simulink library "Chassis_stability_controllers"  (R2024a)
settings: Solver=VariableStepAuto  StartTime=0.0  StopTime=10.0  RelTol=1e-3
undefined symbols (not defined in the file): Ts
settings Model: Creator=Henrique Mesquita  LastModifiedBy=Henrique Mesquita

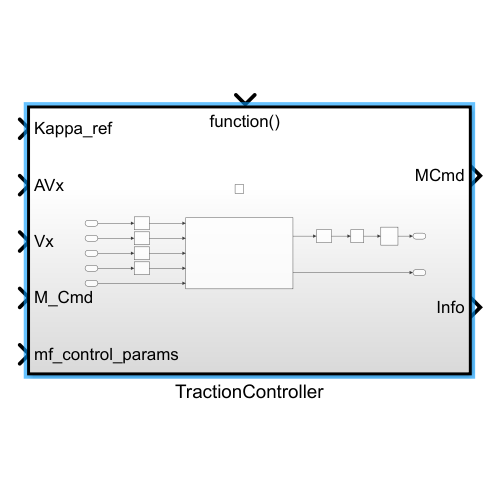
[thumbnail: Simulink's stored preview of the top-level diagram]
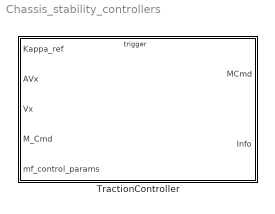
== system Chassis_stability_controllers ==
  TractionController : Subsystem

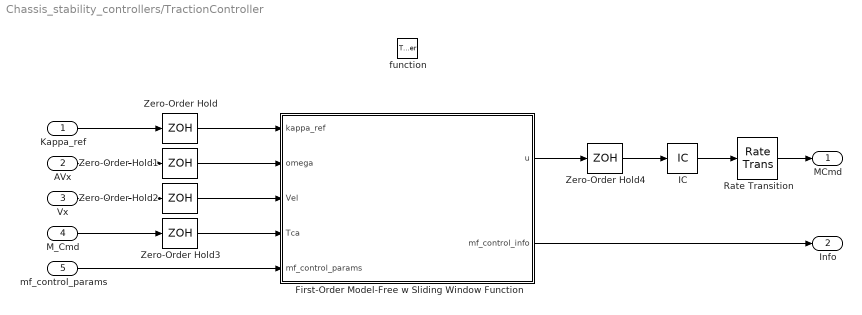
== system Chassis_stability_controllers/TractionController ==
  Kappa_ref : Inport
  AVx : Inport  Port=2
  Vx : Inport  Port=3
  M_Cmd : Inport  Port=4
  mf_control_params : Inport  Port=5
  function : TriggerPort  TriggerType=function-call  VariantControl=(inherit)
  First-Order Model-Free w Sliding Window Function : MATLAB Function  TreatAsAtomicUnit=on  VariantControl=MFC sliding window
  IC : InitialCondition  Value=0
  Rate Transition : RateTransition
  Zero-Order Hold{,1..4} (5 alike) : ZeroOrderHold  SampleTime=Ts
  MCmd : Outport
  Info : Outport  Port=2  OutDataTypeStr=Bus: control_info_bus
  wires:
  Zero-Order Hold3/1 -> First-Order Model-Free w Sliding Window Function/4(Tca)
  Zero-Order Hold/1 -> First-Order Model-Free w Sliding Window Function/1(kappa_ref)
  First-Order Model-Free w Sliding Window Function/1(u) -> Zero-Order Hold4/1
  First-Order Model-Free w Sliding Window Function/2(mf_control_info) -> Info/1
  M_Cmd/1 -> Zero-Order Hold3/1
  Rate Transition/1 -> MCmd/1
  Zero-Order Hold2/1 -> First-Order Model-Free w Sliding Window Function/3(Vel)
  Zero-Order Hold1/1 -> First-Order Model-Free w Sliding Window Function/2(omega)
  Zero-Order Hold4/1 -> IC/1
  IC/1 -> Rate Transition/1
  AVx/1 -> Zero-Order Hold1/1
  Kappa_ref/1 -> Zero-Order Hold/1
  Vx/1 -> Zero-Order Hold2/1
  mf_control_params/1 -> First-Order Model-Free w Sliding Window Function/5(mf_control_params)

== matlab function Chassis_stability_controllers/TractionController/First-Order Model-Free w Sliding Window Function ==
  data: kappa_ref input single; u output single; omega input single; Vel input single; Tca input single; mf_control_info output Bus: BUS_TC_MF_CONTROL_INFO; mf_control_params input Bus: BUS_TC_MF_CONTROL_PARAMS
function [u,mf_control_info] = fcn(kappa_ref, omega, Vel, Tca, mf_control_params)

%%% Definition of persistent variables
persistent u_mem;
persistent kappa_mem;
persistent k_ref_ant;
persistent phi;
persistent alpha_chap;
persistent s_y;
persistent s_u;

%%% Extraction of control parameters
Kp = mf_control_params.Kp;
Td = mf_control_params.Td;
Ts = mf_control_params.Ts;
alpha = mf_control_params.alpha;
N = mf_control_params.N;

%%% Initialization of the persistent values
if (isempty(u_mem)||isempty(kappa_mem)||isempty(k_ref_ant)||isempty(phi)||isempty(alpha_chap)||isempty(s_y)||isempty(s_u))
    
    %%% Initial allocation of the persistent variables
    phi = single(0);
    alpha_chap = alpha;
    u_mem = zeros(1,N+1,'single');
    kappa_mem = zeros(1,N+1,'single');
    k_ref_ant = kappa_ref;
    
    %%% Early calculation and saving of the algebraic estimator coefficients
    T = single(N*Ts);
    i = N-1:-1:1;
    s_y = -6/T^3*[Ts/2*(T-2*N*Ts), Ts*(T-2*i*Ts), Ts/2*(T-2*0*Ts)];
    s_u = -6/T^3*[Ts/2*(T-N*Ts)*(N*Ts), Ts*(T-i*Ts).*(i*Ts), Ts/2*(T-0*Ts)*(0*Ts)];
end

%%% Parameter transformations and definitions
omega = omega*2*pi/60;
Vel = Vel/3.6;
re = single(0.284);
Iw = single(0.8);

%%% Slip and error estimation
dot_yd = (kappa_ref - k_ref_ant) / Ts;
% dot_yd = (3*kappa_ref - 4*k_ref_ant+k_ref_ant_ant) / (2*Ts);
kappa = (omega*re-Vel)/(max([abs(Vel) 1/3.6]));
e = kappa-kappa_ref;

%%% Control signal calculation
ud = Kp*Td/Ts*(kappa-kappa_mem(1));
du = (-phi+dot_yd-Kp*e)/alpha_chap;

%%% Saturation of the control signal
if(du>0)
    du = 0;
elseif (du<-Tca)
    du = -Tca;
end

%%% Block outputs
u = du;
mf_control_info = struct('Phi',phi,'kappa',kappa,'u',du+Tca,'du',du,'e',e,'a',alpha_chap,'ud',ud);

%%% Memory actualization
for i = 0:N-1
    u_mem(N+1-i) = u_mem(N-i);
    kappa_mem(N+1-i) = kappa_mem(N-i);
end
u_mem(1) = du;
kappa_mem(1) = kappa;
k_ref_ant = kappa_ref;
alpha_chap = max([0.01,min([alpha,re/(Iw*max([0.001,abs(Vel)]))])]);

%%% Algebraic Estimation
phi=0;
for i=1:N+1
    phi = phi + s_y(i)*kappa_mem(i) + alpha_chap*s_u(i)*u_mem(i);
end
